simulink model "ControllerWithDelayTest"  (R2017a)
settings: Solver=FixedStepAuto  StartTime=0.0  StopTime=20  FixedStep=0.0025  RelTol=1e-3
undefined symbols (not defined in the file): ki, kp, Standard_Devices, UDP_Protocol
libraries: sldrtlib x2, simulink x1
settings Model: Creator=wangy  LastModifiedBy=wang.yanchao

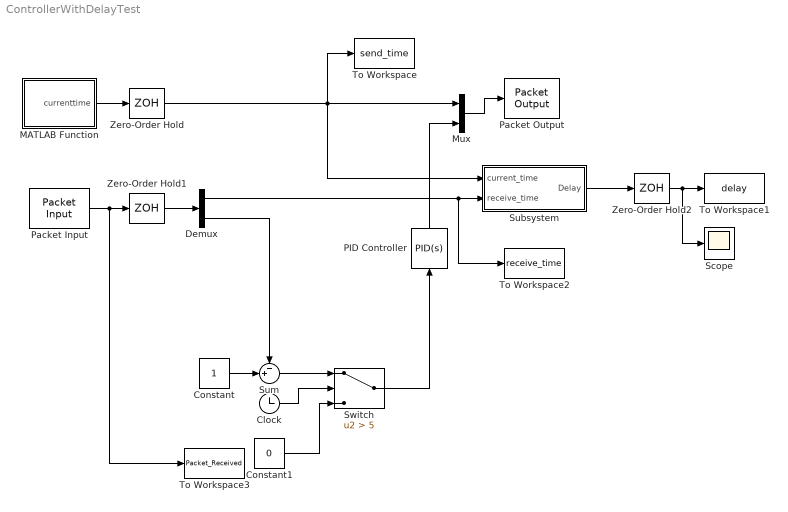
== system ControllerWithDelayTest ==
  Clock : Clock
  Constant : Constant  Priority=1
  Constant1 : Constant  Value=0
  Demux : Demux  Outputs=2
  MATLAB Function : MATLAB Function  Priority=3  TreatAsAtomicUnit=on
  Mux : Mux  Inputs=2
  PID Controller : simulink/Continuous/PID Controller  Controller=PID  TimeDomain=Continuous-time  SampleTime=-1  IntegratorMethod=Forward Euler  FilterMethod=Forward Euler  Form=Parallel  UseFilter=on  ControllerParametersSource=internal  P=kp  I=ki  D=0  N=100  InitialConditionSource=internal  InitialConditionForIntegrator=0  InitialConditionForFilter=0  ExternalReset=none  LimitOutput=off  UpperSaturationLimit=inf  LowerSaturationLimit=-inf  LinearizeAsGain=on  AntiWindupMode=none  Kb=1  TrackingMode=off  Kt=1  PParamMin=[]  PParamMax=[]  IParamMin=[]  IParamMax=[]  DParamMin=[]  DParamMax=[]  NParamMin=[]  NParamMax=[]  KbParamMin=[]  KbParamMax=[]  KtParamMin=[]  KtParamMax=[]  POutMin=[]  POutMax=[]  IOutMin=[]  IOutMax=[]  DOutMin=[]  DOutMax=[]  NOutMin=[]  NOutMax=[]  KbOutMin=[]  KbOutMax=[]  KtOutMin=[]  KtOutMax=[]  IntegratorOutMin=[]  IntegratorOutMax=[]  FilterOutMin=[]  FilterOutMax=[]  SumOutMin=[]  SumOutMax=[]  SumI1OutMin=[]  SumI1OutMax=[]  SumI2OutMin=[]  SumI2OutMax=[]  SumI3OutMin=[]  SumI3OutMax=[]  SumDOutMin=[]  SumDOutMax=[]  SaturationOutMin=[]  SaturationOutMax=[]  IntegratorContinuousStateAttributes=''  IntegratorStateMustResolveToSignalObject=off  IntegratorRTWStateStorageClass=Auto  FilterContinuousStateAttributes=''  FilterStateMustResolveToSignalObject=off  FilterRTWStateStorageClass=Auto  DifferentiatorICPrevScaledInput=0  DifferentiatorOutMin=[]  DifferentiatorOutMax=[]  InitialConditionSetting=State (most efficient)
  Packet Input : sldrtlib/Packet Input  Priority=0  SampleTime=0.0025  MaxMissedTicks=inf  ShowMissedTicks=off  YieldWhenWaiting=off  DrvName=Standard_Devices/UDP_Protocol  DrvAddress=12001  DrvOptions=[424570106 12000]  PacketSize=16  DataTypes='2*double'  ShowReady=off  ShowError=off  PacketID=1  ByteOrder=1  ShowTimestamp=off
      settings: AttributesFormatString=Standard Devices\nUDP Protocol [2EE1h]  SourceProductName=Simulink Desktop Real-Time
  Packet Output : sldrtlib/Packet Output  Priority=4  SampleTime=0.04  MaxMissedTicks=inf  ShowMissedTicks=off  YieldWhenWaiting=off  DrvName=Standard_Devices/UDP_Protocol  DrvAddress=12003  DrvOptions=[424570106 12002]  PacketSize=16  DataTypes='2*double'  ShowReady=off  ShowError=off  PacketID=1  ByteOrder=1  InitialValue=[]  FinalValue=[]
      settings: AttributesFormatString=Standard Devices\nUDP Protocol [2EE3h]  SourceProductName=Simulink Desktop Real-Time
  Scope : Scope
  Subsystem : Subsystem
  Sum : Sum  Priority=2  Inputs=-+|
  Switch : Switch  Criteria=u2 > Threshold  Threshold=5
  To Workspace : ToWorkspace  VariableName=send_time  SaveFormat=Timeseries  SampleTime=-1
  To Workspace1 : ToWorkspace  VariableName=delay  SaveFormat=Timeseries  SampleTime=-1
  To Workspace2 : ToWorkspace  VariableName=receive_time  SaveFormat=Timeseries  SampleTime=-1
  To Workspace3 : ToWorkspace  VariableName=Packet_Received  SaveFormat=Timeseries  SampleTime=-1
  Zero-Order Hold : ZeroOrderHold  SampleTime=-1
  Zero-Order Hold1 : ZeroOrderHold  SampleTime=-1
  Zero-Order Hold2 : ZeroOrderHold  SampleTime=-1
  wires:
  MATLAB Function/1(currenttime) -> Zero-Order Hold/1
  Mux/1 -> Packet Output/1
  Zero-Order Hold/1 -> To Workspace/1, Subsystem/1(current_time), Mux/1
  Constant/1 -> Sum/2
  Packet Input/1 -> To Workspace3/1, Zero-Order Hold1/1
  Zero-Order Hold1/1 -> Demux/1
  Demux/2 -> Sum/1
  Demux/1 -> To Workspace2/1, Subsystem/2(receive_time)
  Subsystem/1(Delay) -> Zero-Order Hold2/1
  Zero-Order Hold2/1 -> Scope/1, To Workspace1/1
  PID Controller/1 -> Mux/2
  Sum/1 -> Switch/1
  Clock/1 -> Switch/2
  Constant1/1 -> Switch/3
  Switch/1 -> PID Controller/1

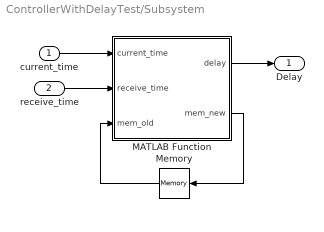
== system ControllerWithDelayTest/Subsystem ==
  current_time : Inport
  receive_time : Inport  Port=2
  MATLAB Function : MATLAB Function  TreatAsAtomicUnit=on
  Memory : Memory
  Delay : Outport
  wires:
  MATLAB Function/1(delay) -> Delay/1
  MATLAB Function/2(mem_new) -> Memory/1
  Memory/1 -> MATLAB Function/3(mem_old)
  current_time/1 -> MATLAB Function/1(current_time)
  receive_time/1 -> MATLAB Function/2(receive_time)

== matlab function ControllerWithDelayTest/Subsystem/MATLAB Function ==
  data: current_time input; delay output; receive_time input; mem_old input; mem_new output
function [delay,mem_new] = fcn(current_time,receive_time,mem_old)
mem_new=0;
if(receive_time~=0)
    mem_new=receive_time;
    if(mem_old==receive_time)
        delay=0; %packet lost
    else
        delay=current_time-receive_time;
        if(delay<0)
            delay=delay+60000;
        end
    end
else
    delay=-50;  %no signal received
end

== matlab function ControllerWithDelayTest/MATLAB Function ==
  data: currenttime output
function currenttime = fun()
coder.extrinsic('current_time');
currenttime=0;
currenttime=current_time();
